simulink model "COM_CalibIMU"  (Simulink 8.6)
settings: Solver=FixedStepDiscrete  StartTime=0.0  StopTime=inf  FixedStep=ComMinSampleTime  RelTol=1e-3
undefined symbols (not defined in the file or in its folder): Gumstix, MPU6050
undefined symbols (not defined in the file): ComMinSampleTime, Ts_AttitudeLoop, Ts_Wifi
settings Model: Creator=Kjenab  LastModifiedBy=arenebiorob  ExtModeTrigDuration=10000
settings SolverCC: PositivePriorityOrder=on
settings DataIOCC: SaveFormat=StructureWithTime
settings OptimizationCC: InitFltsAndDblsToZero=on  OptimizeModelRefInitCode=on  LifeSpan=Inf  SimCompilerOptimization=on
settings DebuggingCC: SaveWithParameterizedLinksMsg=none  UnderspecifiedInitializationDetection=Simplified  MergeDetectMultiDrivingBlocksExec=error  FcnCallInpInsideContextMsg=UseLocalSettings
settings HardwareCC: ProdHWDeviceType=Generic->Unspecified (assume 32-bit Generic)
settings RTWCC: SystemTargetFile=ert.tlc  GenCodeOnly=on  GenerateMakefile=off  TemplateMakefile=ert_default_tmf  PostCodeGenCommand=packNGo(buildInfo, {'packType' 'hierarchical'})  Description=Embedded Coder  RTWCompilerOptimization=on
settings CodeAppCC: IgnoreCustomStorageClasses=off  CustomSymbolStrType=$N$R$M  InternalIdentifier=Classic
settings ERTTargetCC: MultiwordLength=2048  GenerateSampleERTMain=on  ERTCustomFileTemplate=example_file_process.tlc  ConvertIfToSwitch=off  SuppressUnreachableDefaultCases=off

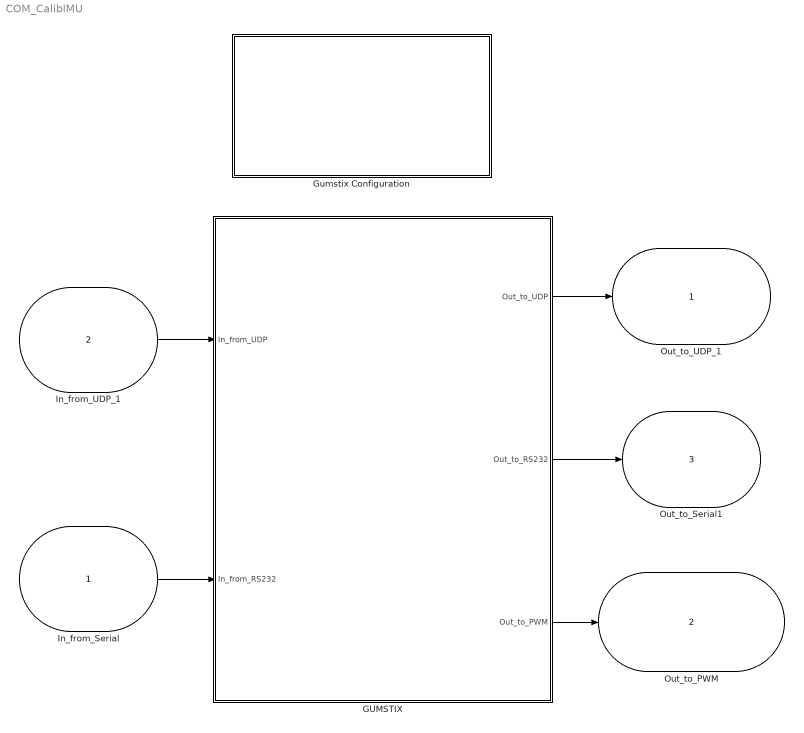
== system COM_CalibIMU ==
  In_from_Serial : Inport  OutDataTypeStr=int16  PortDimensions=Gumstix.RS232.Reception(1).NbData  SampleTime=Gumstix.RS232.Reception(1).SampleTime  mask{RS232_NbData=11, RS232_DataType=int16, RS232_Port=/dev/ttyO0, RS232_BaudRate=115200, RS232_SampleTime=Ts_AttitudeLoop, RS232_BlockingReception=OFF (try to read the n data), RS232_BlockingTimeOut=0.00022, RS232_StreamHeaderReception=1 byte, RS232_StreamHeaderValue=170, RS232_StartProtocol=SendStart -> WaitStart, RS232_StartTimeOut=100, RS232_StartStream=START, RS232_StopProtocol=None, RS232_StopTimeOut=100, RS232_StopStream=STOP}
      mask prompts: RS232_NbData "Number of Received Data"; RS232_DataType "RS232 Data Type"; RS232_Port "Serial Port"; RS232_BaudRate "BaudRate"; RS232_SampleTime "Reception Sample Time [s]"; RS232_BlockingReception "Blocking Reception"; RS232_BlockingTimeOut "Blocking Time Out [s]"; RS232_StreamHeaderReception "Stream Header"; RS232_StreamHeaderValue "Stream header value [0-255]"; RS232_StartProtocol "START Protocols"; RS232_StartTimeOut "Start Stream Waiting TimeOut [ms]"; RS232_StartStream "Start Message"; RS232_StopProtocol "STOP Protocols"; RS232_StopTimeOut "Stop Stream Waiting TimeOut [ms]"; RS232_StopStream "Stop Message"
      mask init:
      | for i=1:1:15
      |     ProcessRS232InportMask_COM(gcb, i);
      | end
      mask Callback RS232_NbData: ProcessRS232InportMask_COM(gcb, 1);
      mask TypeOptions RS232_DataType: double64 | float32 | int32 | unsigned int32 | int16 | unsigned int16 | char8 | unsigned char8
      mask Callback RS232_DataType: ProcessRS232InportMask_COM(gcb, 2);
      mask TypeOptions RS232_Port: /dev/ttyO0 | /dev/ttyO1 | /dev/ttyO2 | /dev/ttyO3 | /dev/ttyO4 | /dev/ttyO5 | /dev/ttyO6 | /dev/ttyO7 | /dev/ttyO8 | /dev/ttyO9 | /dev/ttyO10 | /dev/ttyO11 | /dev/ttyO12 | /dev/ttyO13 | /dev/ttyO14 | /dev/ttyO15 | /dev/ttyUSB0 | /dev/ttyUSB1
      mask Callback RS232_Port: ProcessRS232InportMask_COM(gcb, 3);
      mask TypeOptions RS232_BaudRate: 50 | 75 | 110 | 134 | 150 | 200 | 300 | 600 | 1200 | 1800 | 2400 | 4800 | 9600 | 19200 | 38400 | 57600 | 115200 | 230400 | 460800 | 576000 | 921600 | 1000000 | 1152000 | 1500000 | 2000000 | 2500000 | 3000000 | 3500000 | 4000000
      mask Callback RS232_BaudRate: ProcessRS232InportMask_COM(gcb, 4);
      mask Callback RS232_SampleTime: ProcessRS232InportMask_COM(gcb, 5);
      mask TypeOptions RS232_BlockingReception: ON (wait the n data) | OFF (try to read the n data)
      mask Callback RS232_BlockingReception: ProcessRS232InportMask_COM(gcb, 6);
      mask Callback RS232_BlockingTimeOut: ProcessRS232InportMask_COM(gcb, 7);
      mask TypeOptions RS232_StreamHeaderReception: None | 1 byte
      mask Callback RS232_StreamHeaderReception: ProcessRS232InportMask_COM(gcb, 8);
      mask Callback RS232_StreamHeaderValue: ProcessRS232InportMask_COM(gcb, 9);
      mask TypeOptions RS232_StartProtocol: WaitStart -> SendStart | SendStart -> WaitStart | None
      mask Callback RS232_StartProtocol: ProcessRS232InportMask_COM(gcb, 10);
      mask Callback RS232_StartTimeOut: ProcessRS232InportMask_COM(gcb, 11);
      mask Callback RS232_StartStream: ProcessRS232InportMask_COM(gcb, 12);
      mask TypeOptions RS232_StopProtocol: WaitStop -> SendStop | SendStop -> WaitStop | None
      mask Callback RS232_StopProtocol: ProcessRS232InportMask_COM(gcb, 13);
      mask Callback RS232_StopTimeOut: ProcessRS232InportMask_COM(gcb, 14);
      mask Callback RS232_StopStream: ProcessRS232InportMask_COM(gcb, 15);
      mask Display: Display_RS232_Reception_Block;
  In_from_UDP_1 : Inport  Port=2  OutDataTypeStr=single  PortDimensions=Gumstix.UDP.Reception(1).NbData  SampleTime=Gumstix.UDP.Reception(1).SampleTime  mask{UDP_NbData=18, UDP_DataType=float32, UDP_remoteIPaddress='192.168.137.1', UDP_remotePort=2011, UDP_Interface=wlan0, UDP_localPort=2011, UDP_SampleTime=Ts_Wifi, UDP_BlockingReception=OFF (try to read the n data), UDP_BlockingTimeOut=0.1}
      mask prompts: UDP_NbData "Number of Received Data"; UDP_DataType "UDP Data Type"; UDP_remoteIPaddress "Remote peer's IP address (IPv4)"; UDP_remotePort "Remote peer's Port (1023<port<65536)"; UDP_Interface "Local Interface to use"; UDP_localPort "Local Port (1023<port<65536)"; UDP_SampleTime "Reception Sample Time [s]"; UDP_BlockingReception "Blocking Reception"; UDP_BlockingTimeOut "Blocking Time Out [s]"
      mask init:
      | for i=1:1:8
      |     ProcessUDPInportMask_COM(gcb, i);
      | end
      mask Callback UDP_NbData: ProcessUDPInportMask_COM(gcb, 1);
      mask TypeOptions UDP_DataType: double64 | float32 | int32 | unsigned int32 | int16 | unsigned int16 | char8 | unsigned char8
      mask Callback UDP_DataType: ProcessUDPInportMask_COM(gcb, 2);
      mask Callback UDP_remoteIPaddress: ProcessUDPInportMask_COM(gcb, 3);
      mask Callback UDP_remotePort: ProcessUDPInportMask_COM(gcb, 4);
      mask TypeOptions UDP_Interface: wlan0 | eth0
      mask Callback UDP_Interface: ProcessUDPInportMask_COM(gcb, 5);
      mask Callback UDP_localPort: ProcessUDPInportMask_COM(gcb, 6);
      mask Callback UDP_SampleTime: ProcessUDPInportMask_COM(gcb, 7);
      mask TypeOptions UDP_BlockingReception: ON (wait the n data until the Time Out) | OFF (try to read the n data)
      mask Callback UDP_BlockingReception: ProcessUDPInportMask_COM(gcb, 8);
      mask Callback UDP_BlockingTimeOut: ProcessUDPInportMask_COM(gcb, 9);
      mask Display: Display_UDP_Reception_Block;
  GUMSTIX : Subsystem
  Gumstix Configuration : Subsystem  mask{TimeSynchro=Internal Clock, RS232_InterruptSource=/dev/ttyO0, UDP_InterruptSource=wlan0, PrintfMode=off, FprintfMode=off, TimeLoggerMode=off, PrintfTimeMode=off, FprintfTimeMode=off, TaskingMode=Multi-Tasking, SchedPolicy=SCHED_FIFO     (Real-Time Scheduler), MaxTaskPriority=95, RTsystem=PREEMPT-RT, TargetEndianess=Unspecified (default), TargetWordSize=32 bits (default)}
      mask prompts: TimeSynchro "Time Scheduler"; RS232_InterruptSource "RS232 Interrupt Source"; UDP_InterruptSource "UDP Interrupt Source"; PrintfMode "Verbose mode activated in the Gumstix console"; FprintfMode "Verbose mode logged in a file (onto Gumstix)"; TimeLoggerMode "Time logger mode activated (log time exec of each task)"; PrintfTimeMode "Execution time plotted in the Gumstix console"; FprintfTimeMode "Execution time logged in a file (onto Gumstix)"; TaskingMode "Tasking Mode"; SchedPolicy "Scheduler Policy"; MaxTaskPriority "Maximum Task Priority [1-99]"; RTsystem "RT system"; TargetEndianess "Target Endianess"; TargetWordSize "Target Word Size"
      mask init:
      | for i=1:1:14
      |     ProcessConfigMask_COM(gcb, i);
      | end
      mask TypeOptions TimeSynchro: RS232 Reception | Internal Clock | UDP Reception
      mask Callback TimeSynchro: ProcessConfigMask_COM(gcb, 1);
      mask TypeOptions RS232_InterruptSource: /dev/ttyS0 | /dev/ttyS1 | /dev/ttyS2 | /dev/ttyS3 | /dev/ttyO0 | /dev/ttyO1 | /dev/ttyO2 | /dev/ttyO3
      mask Callback RS232_InterruptSource: ProcessConfigMask_COM(gcb, 2);
      mask TypeOptions UDP_InterruptSource: wlan0 | eth0
      mask Callback UDP_InterruptSource: ProcessConfigMask_COM(gcb, 3);
      mask TypeOptions PrintfMode: off | on
      mask Callback PrintfMode: ProcessConfigMask_COM(gcb, 4);
      mask TypeOptions FprintfMode: off | on
      mask Callback FprintfMode: ProcessConfigMask_COM(gcb, 5);
      mask TypeOptions TimeLoggerMode: off | on
      mask Callback TimeLoggerMode: ProcessConfigMask_COM(gcb, 6);
      mask TypeOptions PrintfTimeMode: off | on
      mask Callback PrintfTimeMode: ProcessConfigMask_COM(gcb, 7);
      mask TypeOptions FprintfTimeMode: off | on
      mask Callback FprintfTimeMode: ProcessConfigMask_COM(gcb, 8);
      mask TypeOptions TaskingMode: Multi-Tasking | Single-Tasking
      mask Callback TaskingMode: ProcessConfigMask_COM(gcb, 9);
      mask TypeOptions SchedPolicy: SCHED_FIFO     (Real-Time Scheduler) | SCHED_RR        (Real-Time Scheduler) | SCHED_OTHER (NO Real-Time Scheduler)
      mask Callback SchedPolicy: ProcessConfigMask_COM(gcb, 10);
      mask Callback MaxTaskPriority: ProcessConfigMask_COM(gcb, 11);
      mask TypeOptions RTsystem: PREEMPT-RT | XENOMAI
      mask Callback RTsystem: ProcessConfigMask_COM(gcb, 12);
      mask TypeOptions TargetEndianess: Unspecified (default) | Little-Endian | Big-Endian
      mask Callback TargetEndianess: ProcessConfigMask_COM(gcb, 13);
      mask TypeOptions TargetWordSize: 32 bits (default) | 64 bits (LLP64) | 64 bits (LP64)
      mask Callback TargetWordSize: ProcessConfigMask_COM(gcb, 14);
      mask Display: image(imread('Configuration_v2.jpg'));
  Out_to_UDP_1 : Outport  OutDataTypeStr=single  PortDimensions=Gumstix.UDP.Emission(1).NbData  SampleTime=Gumstix.UDP.Emission(1).SampleTime  mask{UDP_NbData=22, UDP_DataType=float32, UDP_RemoteIPaddress='192.168.137.1', UDP_RemotePort=2011, UDP_Interface=wlan0, UDP_LocalPort=2011, UDP_SampleTime=Ts_Wifi}
      mask prompts: UDP_NbData "Number of Sent Data"; UDP_DataType "UDP Data Type"; UDP_RemoteIPaddress "remote peer's IP address (IPv4)"; UDP_RemotePort "remote peer's Port (1023<port<65536)"; UDP_Interface "Local Interface to use for UDP"; UDP_LocalPort "Local port to use"; UDP_SampleTime "Emission Sample Time [s]"
      mask init:
      | for i=1:1:7
      |     ProcessUDPOutportMask_COM(gcb, i);
      | end
      mask Callback UDP_NbData: ProcessUDPOutportMask_COM(gcb, 1);
      mask TypeOptions UDP_DataType: double64 | float32 | int32 | unsigned int32 | int16 | unsigned int16 | char8 | unsigned char8
      mask Callback UDP_DataType: ProcessUDPOutportMask_COM(gcb, 2);
      mask Callback UDP_RemoteIPaddress: ProcessUDPOutportMask_COM(gcb, 3);
      mask Callback UDP_RemotePort: ProcessUDPOutportMask_COM(gcb, 4);
      mask TypeOptions UDP_Interface: wlan0 | eth0
      mask Callback UDP_Interface: ProcessUDPOutportMask_COM(gcb, 5);
      mask Callback UDP_LocalPort: ProcessUDPOutportMask_COM(gcb, 6);
      mask Callback UDP_SampleTime: ProcessUDPOutportMask_COM(gcb, 7);
      mask Display: Display_UDP_Emission_Block;
  Out_to_PWM : Outport  Port=2  OutDataTypeStr=uint16  PortDimensions=evalin('base', 'length(Gumstix.PWM.ActivePwm)')  SampleTime=evalin('base', 'Gumstix.PWM.SampleTime')  mask{TimersList=10, PwmFrequency=333, PwmMode=DUTY_CYCLE Mode, ServoMin=10000, ServoMax=20000, PWM_DefaultValue=30, PWM_SampleTime=ComMinSampleTime*3, PWM_KeepAfterStop=on}
      mask prompts: TimersList "Active PWM (example: [8,9,10,11])"; PwmFrequency "PWM Frequency [Hz]"; PwmMode "PWM Mode"; ServoMin "Servo Min Value [tenth's of us]"; ServoMax "Servo Max Value [tenth's of us]"; PWM_DefaultValue "Default Pwm Value"; PWM_SampleTime "Refresh Sample Time [s]"; PWM_KeepAfterStop "Keep Default Pwm Value after program stop"
      mask init:
      | for i=1:1:8
      |     ProcessPWMmask_COM(gcb, i);
      | end
      mask Callback TimersList: ProcessPWMmask_COM(gcb, 1);
      mask Callback PwmFrequency: ProcessPWMmask_COM(gcb, 2);
      mask TypeOptions PwmMode: SERVO Mode | DUTY_CYCLE Mode
      mask Callback PwmMode: ProcessPWMmask_COM(gcb, 3);
      mask Callback ServoMin: ProcessPWMmask_COM(gcb, 4);
      mask Callback ServoMax: ProcessPWMmask_COM(gcb, 5);
      mask Callback PWM_DefaultValue: ProcessPWMmask_COM(gcb, 6);
      mask Callback PWM_SampleTime: ProcessPWMmask_COM(gcb, 7);
      mask Callback PWM_KeepAfterStop: ProcessPWMmask_COM(gcb, 8);
      mask Display: Display_PWM_Block;
  Out_to_Serial1 : Outport  Port=3  OutDataTypeStr=int16  PortDimensions=Gumstix.RS232.Emission(1).NbData  SampleTime=Gumstix.RS232.Emission(1).SampleTime  mask{RS232_NbData=4, RS232_DataType=int16, RS232_Port=/dev/ttyO0, RS232_BaudRate=115200, RS232_SampleTime=Ts_AttitudeLoop, RS232_StreamHeaderReception=1 byte, RS232_StreamHeaderValue=170, RS232_StartProtocol=SendStart -> WaitStart, RS232_StartTimeOut=100, RS232_StartStream=START, RS232_StopProtocol=None, RS232_StopTimeOut=100, RS232_StopStream=STOP}
      mask prompts: RS232_NbData "Number of Sent Data"; RS232_DataType "RS232 Data Type"; RS232_Port "Serial Port"; RS232_BaudRate "BaudRate"; RS232_SampleTime "Sample Time [s]"; RS232_StreamHeaderReception "Stream Header"; RS232_StreamHeaderValue "Stream header value [0-255]"; RS232_StartProtocol "RS232 Start Protocol"; RS232_StartTimeOut "Start Stream Waiting TimeOut [ms]"; RS232_StartStream "Start Message"; RS232_StopProtocol "RS232 Stop Protocol"; RS232_StopTimeOut "Stop Stream Waiting TimeOut [ms]"; RS232_StopStream "Stop Message"
      mask init:
      | for i=1:1:13
      |     ProcessRS232OutportMask_COM(gcb, i);
      | end
      mask Callback RS232_NbData: ProcessRS232OutportMask_COM(gcb, 1);
      mask TypeOptions RS232_DataType: double64 | float32 | int32 | unsigned int32 | int16 | unsigned int16 | char8 | unsigned char8
      mask Callback RS232_DataType: ProcessRS232OutportMask_COM(gcb, 2);
      mask TypeOptions RS232_Port: /dev/ttyO0 | /dev/ttyO1 | /dev/ttyO2 | /dev/ttyO3 | /dev/ttyO4 | /dev/ttyO5 | /dev/ttyO6 | /dev/ttyO7 | /dev/ttyO8 | /dev/ttyO9 | /dev/ttyO10 | /dev/ttyO11 | /dev/ttyO12 | /dev/ttyO13 | /dev/ttyO14 | /dev/ttyO15 | /dev/ttyUSB0 | /dev/ttyUSB1
      mask Callback RS232_Port: ProcessRS232OutportMask_COM(gcb, 3);
      mask TypeOptions RS232_BaudRate: 50 | 75 | 110 | 134 | 150 | 200 | 300 | 600 | 1200 | 1800 | 2400 | 4800 | 9600 | 19200 | 38400 | 57600 | 115200 | 230400 | 460800 | 576000 | 921600 | 1000000 | 1152000 | 1500000 | 2000000 | 2500000 | 3000000 | 3500000 | 4000000
      mask Callback RS232_BaudRate: ProcessRS232OutportMask_COM(gcb, 4);
      mask Callback RS232_SampleTime: ProcessRS232OutportMask_COM(gcb, 5);
      mask TypeOptions RS232_StreamHeaderReception: None | 1 byte
      mask Callback RS232_StreamHeaderReception: ProcessRS232OutportMask_COM(gcb, 6);
      mask Callback RS232_StreamHeaderValue: ProcessRS232OutportMask_COM(gcb, 7);
      mask TypeOptions RS232_StartProtocol: WaitStart -> SendStart | SendStart -> WaitStart | None
      mask Callback RS232_StartProtocol: ProcessRS232OutportMask_COM(gcb, 8);
      mask Callback RS232_StartTimeOut: ProcessRS232OutportMask_COM(gcb, 9);
      mask Callback RS232_StartStream: ProcessRS232OutportMask_COM(gcb, 10);
      mask TypeOptions RS232_StopProtocol: WaitStop -> SendStop | SendStop -> WaitStop | None
      mask Callback RS232_StopProtocol: ProcessRS232OutportMask_COM(gcb, 11);
      mask Callback RS232_StopTimeOut: ProcessRS232OutportMask_COM(gcb, 12);
      mask Callback RS232_StopStream: ProcessRS232OutportMask_COM(gcb, 13);
      mask Display: Display_RS232_Emission_Block;
  wires:
  In_from_UDP_1/1 -> GUMSTIX/1(In_from_UDP)
  In_from_Serial/1 -> GUMSTIX/2(In_from_RS232)
  GUMSTIX/1(Out_to_UDP) -> Out_to_UDP_1/1
  GUMSTIX/3(Out_to_PWM) -> Out_to_PWM/1
  GUMSTIX/2(Out_to_RS232) -> Out_to_Serial1/1

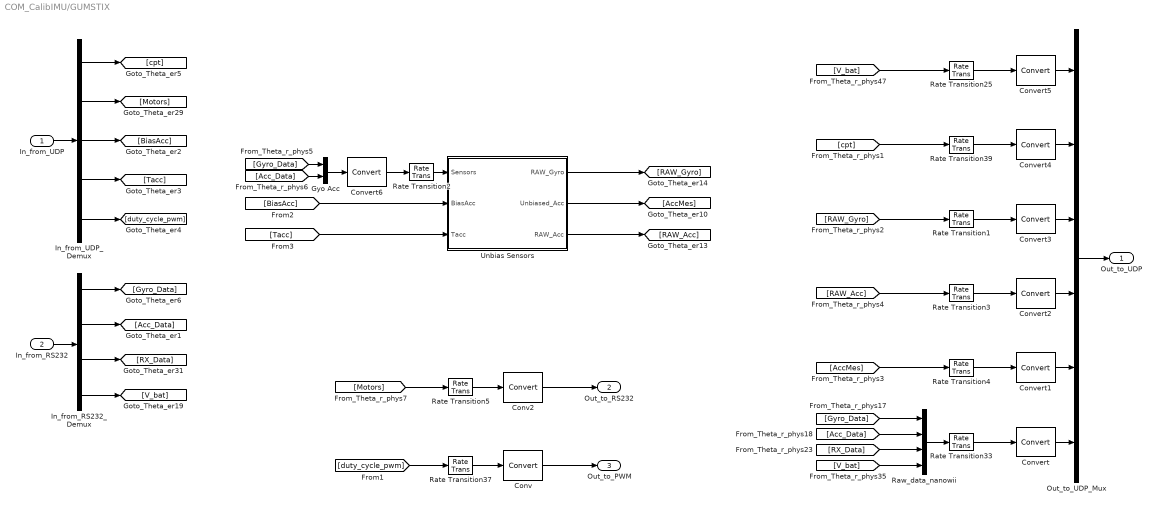
== system COM_CalibIMU/GUMSTIX ==
  In_from_UDP : Inport
  In_from_RS232 : Inport  Port=2
  Conv : DataTypeConversion  RndMeth=Nearest
  Conv2 : DataTypeConversion  RndMeth=Nearest
  Convert{,1..5} (6 alike) : DataTypeConversion  RndMeth=Nearest
  Convert6 : DataTypeConversion
  Gyo Acc : Mux  Inputs=2
  In_from_RS232_Demux : Demux  Outputs=[3 3 4 1]
  In_from_UDP_Demux : Demux  Outputs=[1; 4; 3; 9; 1]
  Out_to_UDP_Mux : Mux  Inputs=[1 1 3 3 3 11]
  Rate Transition{1,3..5,25,33,37,39} (8 alike) : RateTransition  Deterministic=off
  Rate Transition2 : RateTransition  Deterministic=off  OutPortSampleTime=Ts_AttitudeLoop
  Raw_data_nanowii : Mux  Inputs=[3 3 4 1]
  Unbias Sensors : Subsystem
  Out_to_UDP : Outport
  Out_to_RS232 : Outport  Port=2
  Out_to_PWM : Outport  Port=3
  wires:
  Out_to_UDP_Mux/1 -> Out_to_UDP/1
  In_from_UDP/1 -> In_from_UDP_Demux/1
  In_from_RS232_Demux/1 -> [Gyro_Data]
  [Gyro_Data] -> Gyo Acc/1
  [Acc_Data] -> Gyo Acc/2
  In_from_UDP_Demux/1 -> [cpt]
  Gyo Acc/1 -> Convert6/1
  [V_bat] -> Rate Transition25/1
  [cpt] -> Rate Transition39/1
  In_from_RS232_Demux/2 -> [Acc_Data]
  In_from_RS232_Demux/3 -> [RX_Data]
  In_from_RS232_Demux/4 -> [V_bat]
  Rate Transition25/1 -> Convert5/1
  Rate Transition39/1 -> Convert4/1
  [Gyro_Data] -> Raw_data_nanowii/1
  [Acc_Data] -> Raw_data_nanowii/2
  [RX_Data] -> Raw_data_nanowii/3
  [V_bat] -> Raw_data_nanowii/4
  Raw_data_nanowii/1 -> Rate Transition33/1
  Rate Transition33/1 -> Convert/1
  [duty_cycle_pwm] -> Rate Transition37/1
  Rate Transition37/1 -> Conv/1
  Conv/1 -> Out_to_PWM/1
  Rate Transition2/1 -> Unbias Sensors/1(Sensors)
  Unbias Sensors/2(Unbiased_Acc) -> [AccMes]
  Unbias Sensors/1(RAW_Gyro) -> [RAW_Gyro]
  Unbias Sensors/3(RAW_Acc) -> [RAW_Acc]
  [RAW_Gyro] -> Rate Transition1/1
  [RAW_Acc] -> Rate Transition3/1
  [AccMes] -> Rate Transition4/1
  Convert/1 -> Out_to_UDP_Mux/6
  Rate Transition1/1 -> Convert3/1
  Rate Transition3/1 -> Convert2/1
  Rate Transition4/1 -> Convert1/1
  Convert1/1 -> Out_to_UDP_Mux/5
  Convert2/1 -> Out_to_UDP_Mux/4
  Convert3/1 -> Out_to_UDP_Mux/3
  Convert4/1 -> Out_to_UDP_Mux/2
  Convert5/1 -> Out_to_UDP_Mux/1
  [BiasAcc] -> Unbias Sensors/2(BiasAcc)
  [Tacc] -> Unbias Sensors/3(Tacc)
  In_from_RS232/1 -> In_from_RS232_Demux/1
  Convert6/1 -> Rate Transition2/1
  In_from_UDP_Demux/3 -> [BiasAcc]
  In_from_UDP_Demux/4 -> [Tacc]
  In_from_UDP_Demux/5 -> [duty_cycle_pwm]
  In_from_UDP_Demux/2 -> [Motors]
  [Motors] -> Rate Transition5/1
  Rate Transition5/1 -> Conv2/1
  Conv2/1 -> Out_to_RS232/1

== system COM_CalibIMU/Gumstix Configuration ==

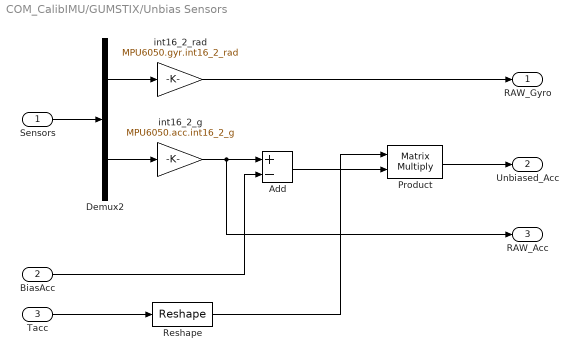
== system COM_CalibIMU/GUMSTIX/Unbias Sensors ==
  Sensors : Inport
  BiasAcc : Inport  Port=2
  Tacc : Inport  Port=3
  Add : Sum  Inputs=+-
  Demux2 : Demux  Outputs=[3 3]
  Product : Product  Multiplication=Matrix(*)  RndMeth=Zero
  Reshape : Reshape  OutputDimensionality=Customize  OutputDimensions=[3,3]
  int16_2_g : Gain  Gain=MPU6050.acc.int16_2_g  OutDataTypeStr=Inherit: Same as input
  int16_2_rad : Gain  Gain=MPU6050.gyr.int16_2_rad  OutDataTypeStr=Inherit: Same as input
  RAW_Gyro : Outport
  Unbiased_Acc : Outport  Port=2
  RAW_Acc : Outport  Port=3
  wires:
  Sensors/1 -> Demux2/1
  int16_2_g/1 -> RAW_Acc/1, Add/1
  Demux2/1 -> int16_2_rad/1
  int16_2_rad/1 -> RAW_Gyro/1
  Demux2/2 -> int16_2_g/1
  Add/1 -> Product/2
  Product/1 -> Unbiased_Acc/1
  BiasAcc/1 -> Add/2
  Reshape/1 -> Product/1
  Tacc/1 -> Reshape/1
